simulink model "Lyapunov_Controller"  (R2025a)
settings: Solver=VariableStepAuto  StartTime=0.0  StopTime=10.0  RelTol=1e-3
settings Model: Creator=hp  LastModifiedBy=hp

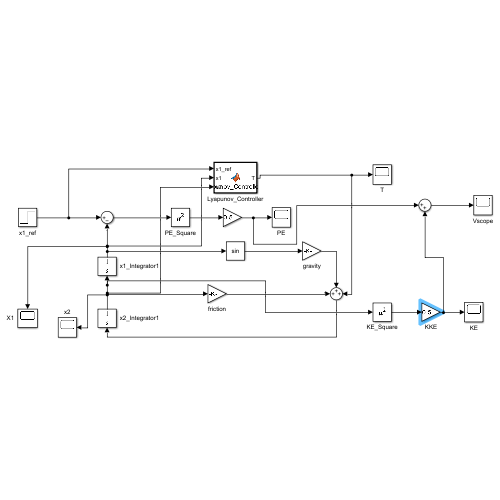
[thumbnail: Simulink's stored preview of the top-level diagram]
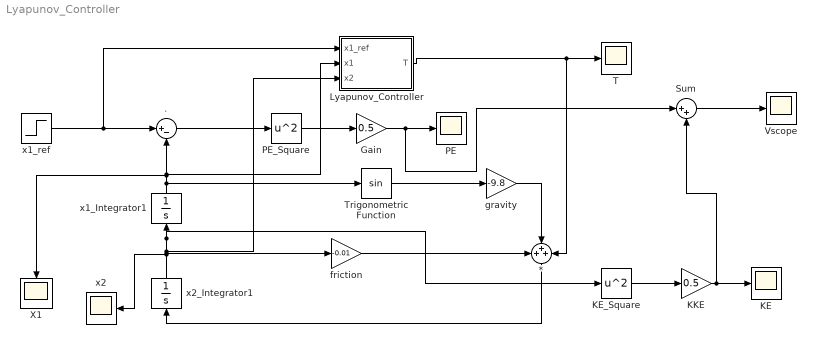
== system Lyapunov_Controller ==
  * : Sum  Inputs=+++
  . : Sum  Inputs=|+-
  Gain : Gain  Gain=0.5
  KE : Scope
      settings: ActiveDisplayYMinimum=-0.016884629016247255  ActiveDisplayYMaximum=0.15196166114622534  DataLoggingVariableName=ScopeData4
  KE_Square : Math  Operator=square
  KKE : Gain  Gain=0.5
  Lyapunov_Controller : MATLAB Function  TreatAsAtomicUnit=on
  PE : Scope
      settings: ActiveDisplayYMinimum=-0.12499971942517332  ActiveDisplayYMaximum=1.1249999688250192  DataLoggingVariableName=ScopeData3
  PE_Square : Math  Operator=square
  Sum : Sum  Inputs=|++
  T : Scope
      settings: ActiveDisplayYMinimum=-0.09585817657034712  ActiveDisplayYMaximum=9.16994675493398  DataLoggingVariableName=ScopeData2
  Trigonometric Function : Trigonometry
  Vscope : Scope
      settings: ActiveDisplayYMinimum=-0.12499948754518364  ActiveDisplayYMaximum=1.1249999430605759  DataLoggingVariableName=ScopeData5
  X1 : Scope
      settings: ActiveDisplayYMinimum=-0.150917494972421  ActiveDisplayYMaximum=1.3582574547517892
  friction : Gain  Gain=-0.01
  gravity : Gain  Gain=-9.8
  x1_Integrator1 : Integrator
  x1_ref : Step  Time=0  SampleTime=0
  x2 : Scope
      settings: ActiveDisplayYMinimum=-0.045941034239891758  ActiveDisplayYMaximum=0.41346930815902588
  x2_Integrator1 : Integrator
  wires:
  x1_ref/1 -> Lyapunov_Controller/1(x1_ref), ./1
  ./1 -> PE_Square/1
  x2_Integrator1/1 -> KE_Square/1, x1_Integrator1/1, Lyapunov_Controller/3(x2), friction/1, x2/1
  x1_Integrator1/1 -> Lyapunov_Controller/2(x1), ./2, X1/1, Trigonometric Function/1
  Trigonometric Function/1 -> gravity/1
  */1 -> x2_Integrator1/1
  friction/1 -> */1
  gravity/1 -> */2
  Lyapunov_Controller/1(T) -> T/1, */3
  KE_Square/1 -> KKE/1
  KKE/1 -> Sum/2, KE/1
  Sum/1 -> Vscope/1
  PE_Square/1 -> Gain/1
  Gain/1 -> Sum/1, PE/1

== matlab function Lyapunov_Controller/Lyapunov_Controller ==
  data: x1_ref input; T output; x1 input; x2 input
function T = Lyapunov_Controller_C(x1_ref,x1,x2)

KPE = 1;
KKE = 1;
KD  = 2;

m = 1;
L = 1;
g = 9.8;
k = 0.01;

e = x1_ref - x1;

T = m*L^2/KKE * (KPE*e - KD*x2) ...
    + m*g*L*sin(x1) ...
    + k*L^2*x2;

end
